simulink model "lsys1_3"  (R2020b)
settings: Solver=VariableStepAuto  StartTime=0.0  StopTime=10.0  RelTol=1e-3
settings Model: Creator=반달  LastModifiedBy=반달
settings DataIOCC: ReturnWorkspaceOutputs=off

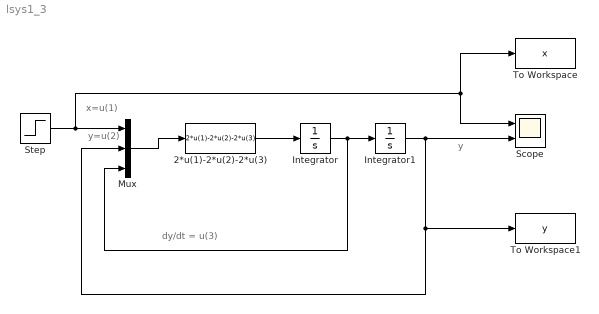
== system lsys1_3 ==
  note: y
  note: dy/dt = u(3)
  note: y=u(2)
  note: x=u(1)
  2*u(1)-2*u(2)-2*u(3) : MATLABFcn  MATLABFcn=2*u(1)-2*u(2)-2*u(3)
  Integrator : Integrator
  Integrator1 : Integrator  InitialCondition=0.25
  Mux : Mux  Inputs=3
  Scope : Scope  NumInputPorts=2
  Step : Step  Time=0.5  SampleTime=0
  To Workspace : ToWorkspace  VariableName=x  SaveFormat=Structure With Time  SampleTime=-1
  To Workspace1 : ToWorkspace  VariableName=y  SaveFormat=Structure With Time  SampleTime=-1
  wires:
  Step/1 -> To Workspace/1, Scope/1, Mux/1
  Mux/1 -> 2*u(1)-2*u(2)-2*u(3)/1
  2*u(1)-2*u(2)-2*u(3)/1 -> Integrator/1
  Integrator/1 -> Mux/3, Integrator1/1
  Integrator1/1 -> Scope/2, To Workspace1/1, Mux/2
